simulink model "step_response_simulation_fopid"  (R2018b)
settings: Solver=VariableStepAuto  StartTime=0.0  StopTime=simStepSimulationTime  FixedStep=4.5e-3  RelTol=1e-6
values from neighbouring files (symbols this model uses):
  C = k_p + k_i/s + (k_d*s)/(1+tau_f*s)    [construct_system_fotfs.m]    (also in evaluate_regulator.m = data.misc(1); generate_optimization_result.m = misc(1))
  G = data.G    [evaluate_regulator.m]    (also in nyqlog_fotf.m = fotf(G); regulator_optimization_genetic_algorithm.m = fotf(G))
  simFractionalFilterOrder = data.simFractionalFilterOrder    [evaluate_regulator.m]    (also in generate_optimization_result.m = 21)
  simFractionalOrderFrequencies = data.simFractionalOrderFrequencies    [evaluate_regulator.m]    (also in generate_optimization_result.m = [1e-5 1e5])
  simStepAmplitude = data.simStepAmplitude    [evaluate_regulator.m]    (also in generate_optimization_result.m = 1)
  simStepSimulationTime = data.simStepSimulationTime    [evaluate_regulator.m]    (also in generate_optimization_result.m = 1)
libraries: cstblocks x2
settings Model: Creator=Raszagal  LastModifiedBy=Raszagal

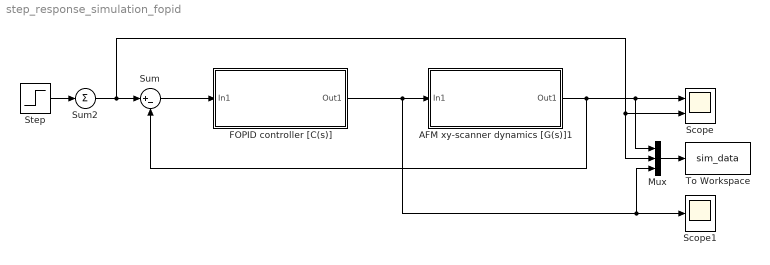
== system step_response_simulation_fopid ==
  AFM xy-scanner dynamics [G(s)]1 : Subsystem  mask{na=G, a=[], nb=[], b=[], ww=simFractionalOrderFrequencies, N=simFractionalFilterOrder, kFilter=Oustaloup filter, T=0}
      mask prompts: na "Orders of the denominator"; a "Coefficients of the denominator"; nb "Orders of the numerator"; b "Coefficients of the numerator"; ww "Interested frequency range [wb wh]"; N "Filter order"; kFilter "Types of the filter"; T "Delay constant T"
      mask init:
      | if isa(na,'fotf'), G=na; 
      | else
      |     if length(na)~=length(a), 
      |        errordlg('Error','Mismatch on the denominator'), 
      |     end
      |     if length(b)~=length(nb), 
      |        errordlg('Error','Mismatch on the numerator'), 
      |     end
      |     G=fotf(a,na,b,nb,T);
      | end
      | switch kFilter, case 1, str='ousta_fod'; 
      |    case 2, str='new_fod'; case 3, str='matsude_fod';
      | end
      | wb=ww(1); wh=ww(2); G1=high_order(G,str,wb,wh,N); [n,m]=size(G1);
      | for i=1:n, for j=1:m, T(i,j)=G(i,j).ioDelay; end, end
      | G1.ioDelay=T;
      mask TypeOptions kFilter: Oustaloup filter | Modified Oustaloup filter
      mask Display: disp('Fractional-order\ntransfer function')
  FOPID controller [C(s)] : Subsystem  mask{na=C, a=[], nb=[], b=[], ww=simFractionalOrderFrequencies, N=simFractionalFilterOrder, kFilter=Oustaloup filter, T=0}
      mask prompts: na "Orders of the denominator"; a "Coefficients of the denominator"; nb "Orders of the numerator"; b "Coefficients of the numerator"; ww "Interested frequency range [wb wh]"; N "Filter order"; kFilter "Types of the filter"; T "Delay constant T"
      mask init: same as step_response_simulation_fopid/AFM xy-scanner dynamics [G(s)]1
      mask TypeOptions kFilter: Oustaloup filter | Modified Oustaloup filter
      mask Display: disp('Fractional-order\ntransfer function')
  Mux : Mux  Inputs=3
  Scope : Scope  NumInputPorts=2
  Scope1 : Scope
  Step : Step  Time=0.01*simStepSimulationTime  After=simStepAmplitude  SampleTime=0
  Sum : Sum  Inputs=|+-
  Sum2 : Sum  Inputs=|+|
  To Workspace : ToWorkspace  VariableName=sim_data  SaveFormat=Timeseries  SampleTime=-1
  wires:
  AFM xy-scanner dynamics [G(s)]1/1(Out1) -> Scope/1, Mux/1, Sum/2
  Sum/1 -> FOPID controller [C(s)]/1(In1)
  FOPID controller [C(s)]/1(Out1) -> AFM xy-scanner dynamics [G(s)]1/1(In1), Scope1/1, Mux/3
  Step/1 -> Sum2/1
  Sum2/1 -> Mux/2, Scope/2, Sum/1
  Mux/1 -> To Workspace/1

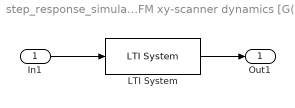
== system step_response_simulation_fopid/AFM xy-scanner dynamics [G(s)]1 ==
  In1 : Inport
  LTI System : cstblocks/LTI System  sys=G1  IC=[]
  Out1 : Outport
  wires:
  LTI System/1 -> Out1/1
  In1/1 -> LTI System/1

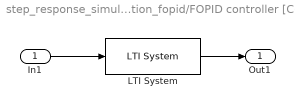
== system step_response_simulation_fopid/FOPID controller [C(s)] ==
  In1 : Inport
  LTI System : cstblocks/LTI System  sys=G1  IC=[]
  Out1 : Outport
  wires:
  LTI System/1 -> Out1/1
  In1/1 -> LTI System/1
